simulink model "Pipeline"  (R2024b)
settings: Solver=VariableStepAuto  StartTime=0.0  StopTime=1000  RelTol=1e-3
model workspace (MAT data in the model file):
  flowR_in_A = 10
  flowR_in_B = 10
  flowR_in_f = 1
  knob = 1
  st_time = 1000
libraries: fl_lib x7, nesl_utility x7, SimscapeFluids_lib x1
(part 2 of 2)

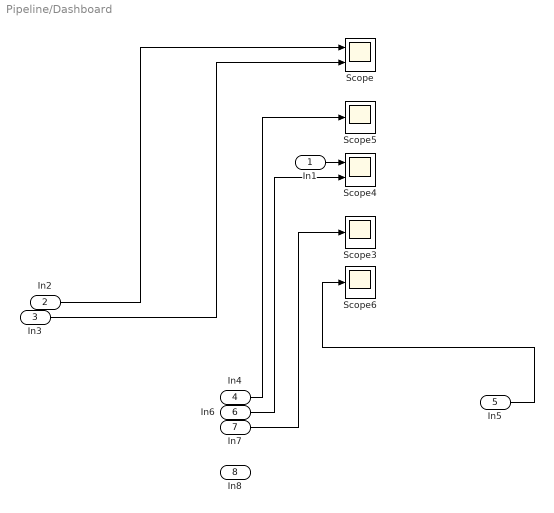
== system Pipeline/Dashboard ==
  In1 : Inport
  In2 : Inport  Port=2
  In3 : Inport  Port=3
  In4 : Inport  Port=4
  In5 : Inport  Port=5
  In6 : Inport  Port=6
  In7 : Inport  Port=7
  In8 : Inport  Port=8
  Scope : Scope  NumInputPorts=2
  Scope3 : Scope
  Scope4 : Scope  NumInputPorts=2
  Scope5 : Scope
  Scope6 : Scope
  wires:
  In5/1 -> Scope6/1
  In2/1 -> Scope/1
  In4/1 -> Scope5/1
  In6/1 -> Scope4/2
  In7/1 -> Scope3/1
  In1/1 -> Scope4/1
  In3/1 -> Scope/2

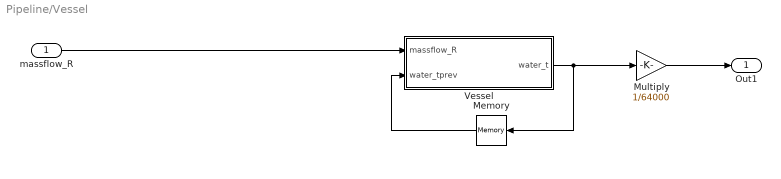
== system Pipeline/Vessel ==
  massflow_R : Inport
  Memory : Memory
  Multiply : Gain  Gain=1/64000
  Vessel : MATLAB Function  TreatAsAtomicUnit=on
  Out1 : Outport
  wires:
  Memory/1 -> Vessel/2(water_tprev)
  Vessel/1(water_t) -> Memory/1, Multiply/1
  Multiply/1 -> Out1/1
  massflow_R/1 -> Vessel/1(massflow_R)

== matlab function Pipeline/Burner ==
  data: Mass_flowR input; flame_T output; p1 input; p2 input; flame_I output; del_p output
function [flame_T, flame_I, del_p] = Burner(Mass_flowR, p1, p2)

    % Parameters
    eta = 0.9;                    % Efficiency
    rho = 1.9;                    % Gas density (kg/m^3)
    Cd = 0.7;                     % Discharge coefficient
    A_nozzle = 7.85e-7;           % Nozzle area in m² (1 mm dia)
    A_flame = 0.00785;
    Hc = 46e6;                    % Calorific value of LPG (J/kg)
    Cp = 1670;                    % Specific heat capacity of combustion gases (J/kg·K)
    T_ambient = 298;              % Ambient temp in Kelvin
    AFR = 15;                     % Air-Fuel Ratio (mass basis)
    sigma = 5.67e-8;              % Stefan-Boltzmann constant (W/m²·K⁴)

    % Pressure difference
    del_p = p1 - p2;

    % Flow velocity through nozzle (optional, not used here)
    velocity = sqrt(complex(2 * (del_p) / rho));

     % Total mass flow of combustion gases
    m_gas = Mass_flowR * (1 + AFR);    % Total mass flow rate of gases (kg/s)

    % Flame Intensity (power) based on fuel mass flow rate
    flame_I = eta * m_gas * Hc;  

   

    % Flame temperature using energy balance:
    %flame_T = eta * Mass_flowR * Hc / (m_gas * Cp *50) + T_ambient;
    flame_T = abs((flame_I / (eta * sigma * A_flame)))^(1/4)/7.5;
end

== matlab function Pipeline/Microprocessor ==
  data: p1 output; flowR_in input; T input; prev_T input; p2 input; prev_p1 input; prev_flowR input
function p1 = microprocessor(flowR_in, T, prev_T, p2, prev_p1,  prev_flowR)
    % MICROPROCESSOR Simulates pressure dynamics in a fluid system
    % using simplified thermodynamic and flow-based modeling.
    %
    % INPUTS:
    %   flowR_in   - Current flow rate [units must be consistent]
    %   prev_flowR - Previous flow rate
    %   T          - Current temperature [K]
    %   prev_T     - Previous temperature [K]
    %   p2         - Downstream pressure [Pa]
    %   prev_p1    - Previous upstream pressure [Pa]
    %
    % OUTPUT:
    %   p1         - Updated upstream pressure (non-dimensional)

    % === Constants ===
    R = 8.314;          % Universal gas constant [J/(mol·K)]
    T1 = 293;           % Reference temperature [K]
    dt = 0.01;          % Time step [s]
    eps_val = 1e-6;     % Small number to prevent division by zero

    % === Safe-guard inputs ===
    if isnan(prev_p1) || isinf(prev_p1)
        prev_p1 = 3000; % Default starting pressure [Pa]
    end
    if isnan(prev_flowR) || isinf(prev_flowR)
        prev_flowR = 0;
    end
    if isnan(prev_T) || isinf(prev_T)
        prev_T = T;
    end

    % Ensure all values are above a small epsilon to avoid zero-division
    flowR_in    = max(flowR_in, eps_val);
    prev_flowR  = max(prev_flowR, eps_val);
    T           = max(T, eps_val);
    prev_T      = max(prev_T, eps_val);
    p2          = max(p2, eps_val);

    % === Compute Derivatives ===
    dv_dt = (flowR_in - prev_flowR) / dt;  % Rate of change of flow
    dT_dt = (T - prev_T) / dt;             % Rate of change of temperature

    % === Compute intermediate terms ===
    P = (flowR_in * dv_dt) / (2 * R * T1);  % Pressure loss term
    Q = (p2 * dT_dt / T) - ...
        ((p2 / flowR_in + (p2 * flowR_in) / (2 * R * T)) * dv_dt); % Thermal + inertial term

    % === Euler Integration to update pressure ===
    dp1_dt = -P * prev_p1 + Q;
    p1 = prev_p1 - dp1_dt * dt;

    % === Normalize to non-dimensional pressure ===
    p1 = p1 / 700000;  % Normalize by reference pressure (e.g., 300000 Pa)

end

== matlab function Pipeline/Vessel/Vessel ==
  data: water_t output; massflow_R input; water_tprev input
function water_t  = Vessel(massflow_R, water_tprev)

H_c = 46e6;
eta = 0.9;
mass_w = 1;
T_ambient = 298;
C_p = 4186;
dt = 0.01;
k = 0.005;

% Validate and initialize previous temperature
if isnan(water_tprev) || isinf(water_tprev)
    water_tprev = T_ambient;  % assign a valid value
end

% Now initialize output variable
water_t = water_tprev;

if massflow_R > 0.01
    dT_dt = eta * massflow_R * H_c / (mass_w * C_p);
    water_t = water_tprev + dT_dt;

else 
    dT_dt = -k * (water_tprev - T_ambient);
    water_t = water_tprev + dT_dt * dt;
end

if isnan(water_t) || isinf(water_t)
    water_t = T_ambient;  % assign a valid value
end

end
